simulink model "dcmotorPID"  (R2013a)
settings: Solver=ode45  StartTime=0.0  StopTime=15  RelTol=1e-3
InitFcn:
  | R = 2.0;    % Ohms
  | L = 0.5;    % Henrys
  | Km = 0.1;   % torque constant
  | Kemf = 0.1;	% back emf constant
  | Kf = 0.2;   % N/m/s
  | J = 0.02;   % kg.m^2/s^2
undefined symbols (not defined in the file): Kd, Ki, Kp
libraries: simulink x2, checkpacklib x1
settings Model: Creator=tloh  LastModifiedBy=IVDL
settings DataIOCC: SignalLoggingSaveFormat=ModelDataLogs
settings OptimizationCC: ExpressionDepthLimit=2147483647
settings DebuggingCC: MultiTaskDSMMsg=warning  MultiTaskCondExecSysMsg=none  FcnCallInpInsideContextMsg=UseLocalSettings  StrictBusMsg=None
settings RTWCC: IncludeERTFirstTime=on
settings GRTTargetCC: CodeReplacementLibrary=None  CombineOutputUpdateFcns=off  CPPClassGenCompliant=on  GRTInterface=on

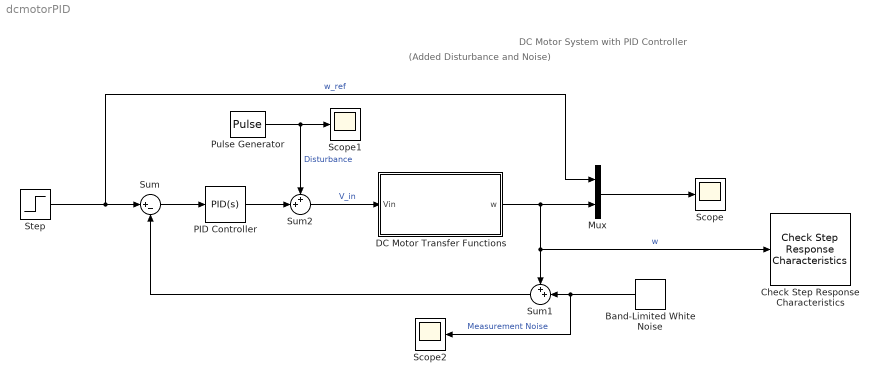
== system dcmotorPID ==
  note: DC Motor System with PID Controller
  note: (Added Disturbance and Noise)
  Band-Limited White Noise : simulink/Sources/Band-Limited White Noise  Cov=[1e-6]  Ts=0.001  seed=[23341]
  Check Step Response Characteristics : checkpacklib/Check Step Response  Characteristics  InstantiateOnLoad=on  enabled=on  stopWhenAssertionFail=off  export=off  ViewDlgPos=[]  OpenViewOnLoad=off  LaunchViewOnOpen=off  TimeUnits=seconds  EnableStepResponseBound=on  InitialValue=0  FinalValue=1  StepTime=1  RiseTime=0.5  PercentRise=90  SettlingTime=1.2  PercentSettling=3  PercentOvershoot=8  PercentUndershoot=3
  DC Motor Transfer Functions : Subsystem
  Mux : Mux  Inputs=2
  PID Controller : simulink/Continuous/PID Controller  Controller=PID  TimeDomain=Continuous-time  SampleTime=1  IntegratorMethod=Forward Euler  FilterMethod=Forward Euler  Form=Parallel  P=Kp  I=Ki  D=Kd  N=100  InitialConditionSource=internal  InitialConditionForIntegrator=0  InitialConditionForFilter=0  ExternalReset=none  LimitOutput=off  UpperSaturationLimit=inf  LowerSaturationLimit=-inf  LinearizeAsGain=off  AntiWindupMode=none  Kb=1  TrackingMode=off  Kt=1  PParamMin=[]  PParamMax=[]  IParamMin=[]  IParamMax=[]  DParamMin=[]  DParamMax=[]  NParamMin=[]  NParamMax=[]  KbParamMin=[]  KbParamMax=[]  KtParamMin=[]  KtParamMax=[]  POutMin=[]  POutMax=[]  IOutMin=[]  IOutMax=[]  DOutMin=[]  DOutMax=[]  NOutMin=[]  NOutMax=[]  KbOutMin=[]  KbOutMax=[]  KtOutMin=[]  KtOutMax=[]  IntegratorOutMin=[]  IntegratorOutMax=[]  FilterOutMin=[]  FilterOutMax=[]  SumOutMin=[]  SumOutMax=[]  SumI1OutMin=[]  SumI1OutMax=[]  SumI2OutMin=[]  SumI2OutMax=[]  SumI3OutMin=[]  SumI3OutMax=[]  SumDOutMin=[]  SumDOutMax=[]  SaturationOutMin=[]  SaturationOutMax=[]  IntegratorContinuousStateAttributes=''  IntegratorStateMustResolveToSignalObject=off  IntegratorRTWStateStorageClass=Auto  FilterContinuousStateAttributes=''  FilterStateMustResolveToSignalObject=off  FilterRTWStateStorageClass=Auto
  Pulse Generator : DiscretePulseGenerator  PulseType=Time based  Amplitude=-2  Period=10  PulseWidth=50  PhaseDelay=5
  Scope : Scope
      settings: ShowLegends=on  TimeRange=15  YMin=-0.2  YMax=1.2
  Scope1 : Scope
      settings: TimeRange=15  YMin=-3  YMax=2
  Scope2 : Scope
      settings: TimeRange=15  YMin=-0.2  YMax=0.15  SaveName=ScopeData2
  Step : Step  SampleTime=0
  Sum : Sum  Inputs=|+-
  Sum1 : Sum  Inputs=++|
  Sum2 : Sum  Inputs=++|
  wires:
  DC Motor Transfer Functions/1(w) -> Sum1/1, Check Step Response Characteristics/1, Mux/2  "w"
  Step/1 -> Mux/1, Sum/1  "w_ref"
  Sum/1 -> PID Controller/1
  Mux/1 -> Scope/1
  Band-Limited White Noise/1 -> Sum1/2, Scope2/1  "Measurement Noise"
  Sum1/1 -> Sum/2
  Sum2/1 -> DC Motor Transfer Functions/1(Vin)  "V_in"
  Pulse Generator/1 -> Sum2/1, Scope1/1  "Disturbance"
  PID Controller/1 -> Sum2/2

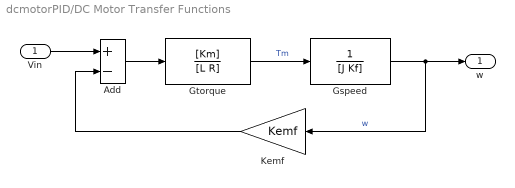
== system dcmotorPID/DC Motor Transfer Functions ==
  Vin : Inport
  Add : Sum  Inputs=+-
  Gspeed : TransferFcn  Denominator=[J Kf]
  Gtorque : TransferFcn  Numerator=[Km]  Denominator=[L R]
  Kemf : Gain  Gain=Kemf
  w : Outport
  wires:
  Add/1 -> Gtorque/1
  Gspeed/1 -> w/1, Kemf/1  "w"
  Vin/1 -> Add/1
  Gtorque/1 -> Gspeed/1  "Tm"
  Kemf/1 -> Add/2
